simulink subsystem "PvtSubSys_HMI"  (R2020b)
settings: Solver=VariableStepAuto  StartTime=0.0  StopTime=10.0  RelTol=1e-3
undefined symbols (not defined in the file): P_HMI_LDW_LKAWarnTime, P_HMI_ObjectTypeFilter, P_HMI_WarnFormLDWReq
libraries: simulink x212, TrueDurationTime x6
(part 5 of 8)

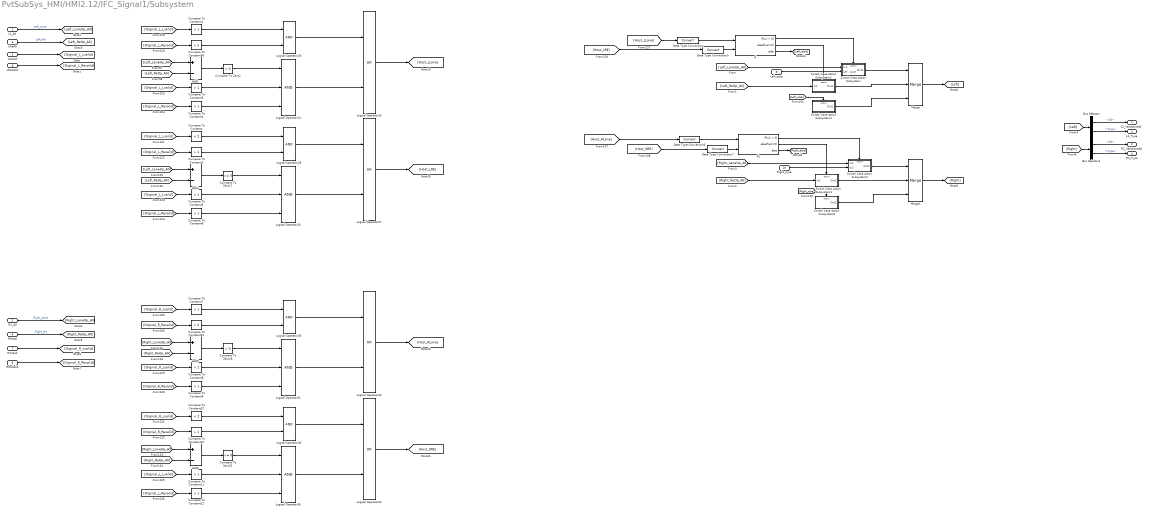
== system PvtSubSys_HMI/HMI2.12/IFC_Signal1/Subsystem ==
  L2_A0 : Inport
  R2_A0 : Inport  Port=2
  LReA0 : Inport  Port=3
  RReA0 : Inport  Port=4
  L2Valid : Inport  Port=5
  LReValid : Inport  Port=6
  R2Valid : Inport  Port=7
  RReValid : Inport  Port=8
  Left_type : Inport  Port=9
  Right_type : Inport  Port=10
  Add{1,4..6} (4 alike) : Sum  Inputs=+-
  Bus Selector : BusSelector  OutputSignals=A0,Type
  Bus Selector1 : BusSelector  OutputSignals=A0,Type
  Compare To Constant{,23,37..38} (4 alike) : simulink/Logic and Bit Operations/Compare To Constant  relop=<  const=2  OutDataTypeStr=boolean
  Compare To Constant{1..12} (12 alike) : simulink/Logic and Bit Operations/Compare To Constant  relop=>  const=1  OutDataTypeStr=boolean
  Compare To Zero17 : simulink/Logic and Bit Operations/Compare To Zero  relop=>=  OutDataTypeStr=boolean
  Compare To Zero2 : simulink/Logic and Bit Operations/Compare To Zero  relop=<  OutDataTypeStr=boolean
  Compare To Zero23 : simulink/Logic and Bit Operations/Compare To Zero  relop=<=  OutDataTypeStr=boolean
  Compare To Zero26 : simulink/Logic and Bit Operations/Compare To Zero  relop=>  OutDataTypeStr=boolean
  Data Type Conversion{,5..7} (4 alike) : DataTypeConversion
  If : If  NumInputs=2  ElseIfExpressions=u2>0
  If1 : If  NumInputs=2  ElseIfExpressions=u2>0
  Logical Operator{24,30..31,36} (4 alike) : Logic  Inputs=3  AllPortsSameDT=off  OutDataTypeStr=boolean
  Logical Operator{25,27,32..33} (4 alike) : Logic  Operator=OR  AllPortsSameDT=off  OutDataTypeStr=boolean
  Logical Operator{28..29,34..35} (4 alike) : Logic  AllPortsSameDT=off  OutDataTypeStr=boolean
  Merge : Merge  Inputs=3
  Merge1 : Merge  Inputs=3
  Switch Case Action Subsystem : Subsystem  TreatAsAtomicUnit=on
  Switch Case Action Subsystem1 : Subsystem  TreatAsAtomicUnit=on
  Switch Case Action Subsystem2 : Subsystem  TreatAsAtomicUnit=on
  Switch Case Action Subsystem3 : Subsystem  TreatAsAtomicUnit=on
  Switch Case Action Subsystem4 : Subsystem  TreatAsAtomicUnit=on
  Switch Case Action Subsystem5 : Subsystem  TreatAsAtomicUnit=on
  L2_ValidLaneA0 : Outport
  R2_ValidLaneA0 : Outport  Port=2
  L2_Type : Outport  Port=3
  R2_Type : Outport  Port=4
  wires:
  Bus Selector1/1 -> R2_ValidLaneA0/1  "<A0>"
  Bus Selector1/2 -> R2_Type/1  "<Type>"
  [Right] -> Bus Selector1/1
  Bus Selector/2 -> L2_Type/1  "<Type>"
  Bus Selector/1 -> L2_ValidLaneA0/1  "<A0>"
  [Left] -> Bus Selector/1
  Logical Operator33/1 -> [Host_RRE]
  Compare To Constant7/1 -> Logical Operator35/1
  Add5/1 -> Compare To Zero26/1
  Compare To Constant37/1 -> Logical Operator34/1
  [Orginal_L_Lvalid] -> Compare To Constant/1
  [Orginal_R_Lvalid] -> Compare To Constant7/1
  Compare To Constant3/1 -> Logical Operator24/2
  [Orginal_L_Revalid] -> Compare To Constant12/1
  Compare To Constant9/1 -> Logical Operator31/3
  Add6/1 -> Compare To Zero23/1
  Compare To Constant6/1 -> Logical Operator30/3
  Compare To Constant38/1 -> Logical Operator29/2
  Logical Operator32/1 -> [Host_RLane]
  Compare To Constant23/1 -> Logical Operator35/2
  Compare To Constant/1 -> Logical Operator28/1
  [Orginal_R_Lvalid] -> Compare To Constant8/1
  Logical Operator31/1 -> Logical Operator32/2
  [Right_LaneOp_A0] -> Add5/1
  Logical Operator34/1 -> Logical Operator33/1
  [Orginal_R_Revalid] -> Compare To Constant23/1
  [Right_ReOp_A0] -> Add6/2
  Logical Operator36/1 -> Logical Operator33/2
  [Right_LaneOp_A0] -> Add6/1
  [Orginal_R_Lvalid] -> Compare To Constant37/1
  [Orginal_L_Lvalid] -> Compare To Constant11/1
  [Orginal_R_Revalid] -> Compare To Constant9/1
  Compare To Constant11/1 -> Logical Operator36/2
  Compare To Constant12/1 -> Logical Operator36/3
  Compare To Constant10/1 -> Logical Operator34/2
  [Orginal_R_Revalid] -> Compare To Constant10/1
  Compare To Constant1/1 -> Logical Operator29/1
  [Left_LaneOp_A0] -> Add1/1
  Compare To Constant5/1 -> Logical Operator30/2
  Logical Operator27/1 -> [Host_LRE]
  Compare To Zero23/1 -> Logical Operator36/1
  Compare To Zero17/1 -> Logical Operator30/1
  Compare To Constant8/1 -> Logical Operator31/2
  [Orginal_L_Revalid] -> Compare To Constant2/1
  [Right_ReOp_A0] -> Add5/2
  Logical Operator25/1 -> [Host_LLane]
  Compare To Constant2/1 -> Logical Operator28/2
  Logical Operator30/1 -> Logical Operator27/2
  Logical Operator35/1 -> Logical Operator32/1
  [Orginal_L_Lvalid] -> Compare To Constant1/1
  [Orginal_L_Revalid] -> Compare To Constant6/1
  Logical Operator28/1 -> Logical Operator27/1
  Compare To Zero26/1 -> Logical Operator31/1
  [Orginal_L_Revalid] -> Compare To Constant38/1
  Add4/1 -> Compare To Zero17/1
  [Left_ReOp_A0] -> Add4/2
  [Left_LaneOp_A0] -> Add4/1
  Logical Operator24/1 -> Logical Operator25/2
  Logical Operator29/1 -> Logical Operator25/1
  [Orginal_L_Revalid] -> Compare To Constant4/1
  Add1/1 -> Compare To Zero2/1
  [Left_ReOp_A0] -> Add1/2
  [Orginal_L_Lvalid] -> Compare To Constant5/1
  Compare To Zero2/1 -> Logical Operator24/1
  [Orginal_L_Lvalid] -> Compare To Constant3/1
  Compare To Constant4/1 -> Logical Operator24/3
  Switch Case Action Subsystem5/1(Out1) -> Merge1/3
  If1/1 -> Switch Case Action Subsystem2/Action
  [Host_RLane] -> Data Type Conversion6/1
  Switch Case Action Subsystem4/1(Out1) -> Merge/3
  Data Type Conversion7/1 -> If1/2
  [Host_LLane] -> Data Type Conversion/1
  Switch Case Action Subsystem3/1(Out1) -> Merge1/2
  Switch Case Action Subsystem1/1(Out1) -> Merge/2
  If1/2 -> Switch Case Action Subsystem3/Action
  Switch Case Action Subsystem2/1(Out1) -> Merge1/1
  Data Type Conversion/1 -> If/1
  [Host_LRE] -> Data Type Conversion5/1
  If/3 -> [Left_else]
  [Host_RRE] -> Data Type Conversion7/1
  [Right_else] -> Switch Case Action Subsystem5/Action
  Switch Case Action Subsystem/1(Out1) -> Merge/1
  Data Type Conversion6/1 -> If1/1
  If/2 -> Switch Case Action Subsystem1/Action
  If/1 -> Switch Case Action Subsystem/Action
  Data Type Conversion5/1 -> If/2
  If1/3 -> [Right_else]
  [Left_else] -> Switch Case Action Subsystem4/Action
  L2Valid/1 -> [Orginal_L_Lvalid]
  LReValid/1 -> [Orginal_L_Revalid]
  L2_A0/1 -> [Left_LaneOp_A0]  "Left_Lane"
  LReA0/1 -> [Left_ReOp_A0]  "Left_Re"
  R2_A0/1 -> [Right_LaneOp_A0]  "Right_Lane"
  RReA0/1 -> [Right_ReOp_A0]  "Right_Re"
  R2Valid/1 -> [Orginal_R_Lvalid]
  RReValid/1 -> [Orginal_R_Revalid]
  [Left_LaneOp_A0] -> Switch Case Action Subsystem/1(In1)
  [Left_ReOp_A0] -> Switch Case Action Subsystem1/1(In1)
  [Right_LaneOp_A0] -> Switch Case Action Subsystem2/1(In1)
  [Right_ReOp_A0] -> Switch Case Action Subsystem3/1(In1)
  Merge/1 -> [Left]
  Merge1/1 -> [Right]
  Left_type/1 -> Switch Case Action Subsystem/2(Left_type)
  Right_type/1 -> Switch Case Action Subsystem2/2(In2)

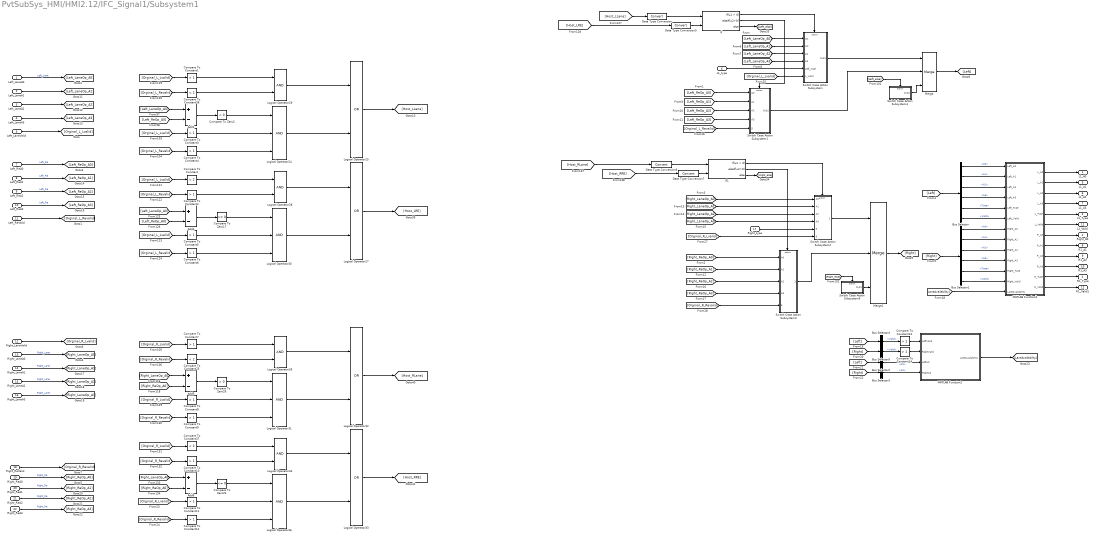
== system PvtSubSys_HMI/HMI2.12/IFC_Signal1/Subsystem1 ==
  Left_LaneA0 : Inport
  Left_LaneA1 : Inport  Port=2
  Left_LaneA2 : Inport  Port=3
  Left_LaneA3 : Inport  Port=4
  Left_LaneValid : Inport  Port=5
  L1_type : Inport  Port=6
  Left_ReA0 : Inport  Port=7
  Left_ReA1 : Inport  Port=8
  Left_ReA2 : Inport  Port=9
  Left_ReA3 : Inport  Port=10
  Left_ReValid : Inport  Port=11
  Right_LaneValid : Inport  Port=12
  Right_LaneA0 : Inport  Port=13
  Right_LaneA1 : Inport  Port=14
  Right_LaneA2 : Inport  Port=15
  Right_LaneA3 : Inport  Port=16
  Right_type : Inport  Port=17
  Right_ReValid : Inport  Port=18
  Right_ReA0 : Inport  Port=19
  Right_ReA1 : Inport  Port=20
  Right_ReA2 : Inport  Port=21
  Right_ReA3 : Inport  Port=22
  Add{1,4..6} (4 alike) : Sum  Inputs=+-
  Bus Selector : BusSelector  OutputSignals=A0,A1,A2,A3,Type,Valid
  Bus Selector1 : BusSelector  OutputSignals=A0,A1,A2,A3,Type,Valid
  Bus Selector2 : BusSelector  OutputSignals=A0
  Bus Selector3 : BusSelector  OutputSignals=A0
  Bus Selector4 : BusSelector  OutputSignals=Valid
  Bus Selector5 : BusSelector  OutputSignals=Valid
  Compare To Constant{,23,37..38} (4 alike) : simulink/Logic and Bit Operations/Compare To Constant  relop=<  const=2  OutDataTypeStr=boolean
  Compare To Constant{1..14} (14 alike) : simulink/Logic and Bit Operations/Compare To Constant  relop=>  const=1  OutDataTypeStr=boolean
  Compare To Zero17 : simulink/Logic and Bit Operations/Compare To Zero  relop=>=  OutDataTypeStr=boolean
  Compare To Zero2 : simulink/Logic and Bit Operations/Compare To Zero  relop=<  OutDataTypeStr=boolean
  Compare To Zero23 : simulink/Logic and Bit Operations/Compare To Zero  relop=<=  OutDataTypeStr=boolean
  Compare To Zero26 : simulink/Logic and Bit Operations/Compare To Zero  relop=>  OutDataTypeStr=boolean
  Data Type Conversion{,5..7} (4 alike) : DataTypeConversion
  If : If  NumInputs=2  ElseIfExpressions=u2>0
  If1 : If  NumInputs=2  ElseIfExpressions=u2>0
  Logical Operator{24,30..31,36} (4 alike) : Logic  Inputs=3  AllPortsSameDT=off  OutDataTypeStr=boolean
  Logical Operator{25,27,32..33} (4 alike) : Logic  Operator=OR  AllPortsSameDT=off  OutDataTypeStr=boolean
  Logical Operator{28..29,34..35} (4 alike) : Logic  AllPortsSameDT=off  OutDataTypeStr=boolean
  MATLAB Function2 : MATLAB Function  TreatAsAtomicUnit=on
  MATLAB Function3 : MATLAB Function  TreatAsAtomicUnit=on
  Merge : Merge  Inputs=3
  Merge1 : Merge  Inputs=3
  Switch Case Action Subsystem : Subsystem  TreatAsAtomicUnit=on
  Switch Case Action Subsystem1 : Subsystem  TreatAsAtomicUnit=on
  Switch Case Action Subsystem2 : Subsystem  TreatAsAtomicUnit=on
  Switch Case Action Subsystem3 : Subsystem  TreatAsAtomicUnit=on
  Switch Case Action Subsystem4 : Subsystem  TreatAsAtomicUnit=on
  Switch Case Action Subsystem5 : Subsystem  TreatAsAtomicUnit=on
  L1_A0 : Outport
  Right_A0 : Outport  Port=2
  L1_Type : Outport  Port=3
  R1_Type : Outport  Port=4
  L1_A1 : Outport  Port=5
  L1_A2 : Outport  Port=6
  L1_A3 : Outport  Port=7
  R1_A1 : Outport  Port=8
  R1_A2 : Outport  Port=9
  R1_A3 : Outport  Port=10
  L1_Valid : Outport  Port=11
  R1_Valid1 : Outport  Port=12
  wires:
  Bus Selector1/6 -> MATLAB Function3/12(Right_Valid)  "<Valid>"
  [Orginal_R_Revalid] -> Switch Case Action Subsystem3/5(Valid)
  [Orginal_R_Lvalid] -> Switch Case Action Subsystem2/6(Valid)
  [Orginal_L_Revalid] -> Switch Case Action Subsystem1/5(LRE_Valid)
  [Orginal_L_Lvalid] -> Switch Case Action Subsystem/6(L_Valid)
  Bus Selector/6 -> MATLAB Function3/6(Left_Valid)  "<Valid>"
  Compare To Constant14/1 -> MATLAB Function2/2(RightValid)
  Bus Selector5/1 -> Compare To Constant14/1  "<Valid>"
  [Right] -> Bus Selector5/1
  Compare To Constant13/1 -> MATLAB Function2/1(LeftValid)
  Bus Selector4/1 -> Compare To Constant13/1  "<Valid>"
  [Left] -> Bus Selector4/1
  Bus Selector3/1 -> MATLAB Function2/4(RightA0)  "<A0>"
  [Right] -> Bus Selector3/1
  Bus Selector2/1 -> MATLAB Function2/3(LeftA0)  "<A0>"
  [Left] -> Bus Selector2/1
  MATLAB Function3/12(R_Valid) -> R1_Valid1/1
  MATLAB Function3/6(L_Valid) -> L1_Valid/1
  MATLAB Function2/1(LaneAvailability) -> [LaneAvailability]
  MATLAB Function3/10(R_A3) -> R1_A3/1
  MATLAB Function3/9(R_A2) -> R1_A2/1
  MATLAB Function3/8(R_A1) -> R1_A1/1
  MATLAB Function3/4(L_A3) -> L1_A3/1
  MATLAB Function3/3(L_A2) -> L1_A2/1
  MATLAB Function3/2(L_A1) -> L1_A1/1
  Bus Selector1/4 -> MATLAB Function3/10(Right_A3)  "<A3>"
  Bus Selector1/3 -> MATLAB Function3/9(Right_A2)  "<A2>"
  Bus Selector1/2 -> MATLAB Function3/8(Right_A1)  "<A1>"
  Bus Selector/4 -> MATLAB Function3/4(Left_A3)  "<A3>"
  Bus Selector/3 -> MATLAB Function3/3(Left_A2)  "<A2>"
  Bus Selector/2 -> MATLAB Function3/2(Left_A1)  "<A1>"
  [Right_ReOp_A3] -> Switch Case Action Subsystem3/4(A3)
  [Right_ReOp_A2] -> Switch Case Action Subsystem3/3(A2)
  [Right_ReOp_A1] -> Switch Case Action Subsystem3/2(A1)
  [Right_LaneOp_A3] -> Switch Case Action Subsystem2/4(A3)
  [Right_LaneOp_A2] -> Switch Case Action Subsystem2/3(A2)
  [Right_LaneOp_A1] -> Switch Case Action Subsystem2/2(A1)
  Right_type/1 -> Switch Case Action Subsystem2/5(Right_type)
  [Left_ReOp_A3] -> Switch Case Action Subsystem1/4(A3)
  [Left_ReOp_A2] -> Switch Case Action Subsystem1/3(A2)
  [Left_ReOp_A1] -> Switch Case Action Subsystem1/2(A1)
  [Left_LaneOp_A3] -> Switch Case Action Subsystem/4(A3)
  [Left_LaneOp_A2] -> Switch Case Action Subsystem/3(A2)
  [Left_LaneOp_A1] -> Switch Case Action Subsystem/2(In2)
  L1_type/1 -> Switch Case Action Subsystem/5(Left_type)
  Right_ReA1/1 -> [Right_ReOp_A1]  "Right_Re"
  Right_ReA2/1 -> [Right_ReOp_A2]  "Right_Re"
  Right_ReA3/1 -> [Right_ReOp_A3]  "Right_Re"
  Right_LaneA3/1 -> [Right_LaneOp_A3]  "Right_Lane"
  Right_LaneA2/1 -> [Right_LaneOp_A2]  "Right_Lane"
  Right_LaneA1/1 -> [Right_LaneOp_A1]  "Right_Lane"
  Left_ReA1/1 -> [Left_ReOp_A1]  "Left_Re"
  Left_ReA2/1 -> [Left_ReOp_A2]  "Left_Re"
  Left_ReA3/1 -> [Left_ReOp_A3]  "Left_Re"
  Left_LaneA3/1 -> [Left_LaneOp_A3]
  Left_LaneA2/1 -> [Left_LaneOp_A2]
  Left_LaneA1/1 -> [Left_LaneOp_A1]
  Logical Operator33/1 -> [Host_RRE]
  Compare To Constant7/1 -> Logical Operator35/1
  Add5/1 -> Compare To Zero26/1
  Compare To Constant37/1 -> Logical Operator34/1
  [Orginal_L_Lvalid] -> Compare To Constant/1
  [Orginal_R_Lvalid] -> Compare To Constant7/1
  Compare To Constant3/1 -> Logical Operator24/2
  [Orginal_R_Revalid] -> Compare To Constant12/1
  Compare To Constant9/1 -> Logical Operator31/3
  Add6/1 -> Compare To Zero23/1
  Compare To Constant6/1 -> Logical Operator30/3
  Compare To Constant38/1 -> Logical Operator29/2
  Logical Operator32/1 -> [Host_RLane]
  Compare To Constant23/1 -> Logical Operator35/2
  Compare To Constant/1 -> Logical Operator28/1
  [Orginal_R_Lvalid] -> Compare To Constant8/1
  Logical Operator31/1 -> Logical Operator32/2
  [Right_LaneOp_A0] -> Add5/1
  Logical Operator34/1 -> Logical Operator33/1
  [Orginal_R_Revalid] -> Compare To Constant23/1
  [Right_ReOp_A0] -> Add6/2
  Logical Operator36/1 -> Logical Operator33/2
  [Right_LaneOp_A0] -> Add6/1
  [Orginal_R_Lvalid] -> Compare To Constant37/1
  [Orginal_R_Lvalid] -> Compare To Constant11/1
  [Orginal_R_Revalid] -> Compare To Constant9/1
  Compare To Constant11/1 -> Logical Operator36/2
  Compare To Constant12/1 -> Logical Operator36/3
  Compare To Constant10/1 -> Logical Operator34/2
  [Orginal_R_Revalid] -> Compare To Constant10/1
  Compare To Constant1/1 -> Logical Operator29/1
  [Left_LaneOp_A0] -> Add1/1
  Compare To Constant5/1 -> Logical Operator30/2
  Logical Operator27/1 -> [Host_LRE]
  Compare To Zero23/1 -> Logical Operator36/1
  Compare To Zero17/1 -> Logical Operator30/1
  Compare To Constant8/1 -> Logical Operator31/2
  [Orginal_L_Revalid] -> Compare To Constant2/1
  [Right_ReOp_A0] -> Add5/2
  Logical Operator25/1 -> [Host_LLane]
  Compare To Constant2/1 -> Logical Operator28/2
  Logical Operator30/1 -> Logical Operator27/2
  Logical Operator35/1 -> Logical Operator32/1
  [Orginal_L_Lvalid] -> Compare To Constant1/1
  [Orginal_L_Revalid] -> Compare To Constant6/1
  Logical Operator28/1 -> Logical Operator27/1
  Compare To Zero26/1 -> Logical Operator31/1
  [Orginal_L_Revalid] -> Compare To Constant38/1
  Add4/1 -> Compare To Zero17/1
  [Left_ReOp_A0] -> Add4/2
  [Left_LaneOp_A0] -> Add4/1
  Logical Operator24/1 -> Logical Operator25/2
  Logical Operator29/1 -> Logical Operator25/1
  [Orginal_L_Revalid] -> Compare To Constant4/1
  Add1/1 -> Compare To Zero2/1
  [Left_ReOp_A0] -> Add1/2
  [Orginal_L_Lvalid] -> Compare To Constant5/1
  Compare To Zero2/1 -> Logical Operator24/1
  [Orginal_L_Lvalid] -> Compare To Constant3/1
  Compare To Constant4/1 -> Logical Operator24/3
  Switch Case Action Subsystem5/1(Out1) -> Merge1/3
  If1/1 -> Switch Case Action Subsystem2/Action
  [Host_RLane] -> Data Type Conversion6/1
  Switch Case Action Subsystem4/1(Out2) -> Merge/3
  Data Type Conversion7/1 -> If1/2
  [Host_LLane] -> Data Type Conversion/1
  Switch Case Action Subsystem3/1(Out1) -> Merge1/2
  Switch Case Action Subsystem1/1(Out2) -> Merge/2
  If1/2 -> Switch Case Action Subsystem3/Action
  Switch Case Action Subsystem2/1(Out1) -> Merge1/1
  Data Type Conversion/1 -> If/1
  [Host_LRE] -> Data Type Conversion5/1
  If/3 -> [Left_else]
  [Host_RRE] -> Data Type Conversion7/1
  [Right_else] -> Switch Case Action Subsystem5/Action
  Switch Case Action Subsystem/1(Out1) -> Merge/1
  Data Type Conversion6/1 -> If1/1
  If/2 -> Switch Case Action Subsystem1/Action
  If/1 -> Switch Case Action Subsystem/Action
  Data Type Conversion5/1 -> If/2
  If1/3 -> [Right_else]
  [Left_else] -> Switch Case Action Subsystem4/Action
  Left_LaneValid/1 -> [Orginal_L_Lvalid]
  Left_ReValid/1 -> [Orginal_L_Revalid]
  Left_LaneA0/1 -> [Left_LaneOp_A0]  "Left_Lane"
  Left_ReA0/1 -> [Left_ReOp_A0]  "Left_Re"
  Right_LaneA0/1 -> [Right_LaneOp_A0]  "Right_Lane"
  Right_ReA0/1 -> [Right_ReOp_A0]  "Right_Re"
  Right_LaneValid/1 -> [Orginal_R_Lvalid]
  Right_ReValid/1 -> [Orginal_R_Revalid]
  [Left_LaneOp_A0] -> Switch Case Action Subsystem/1(In1)
  [Left_ReOp_A0] -> Switch Case Action Subsystem1/1(A0)
  [Right_LaneOp_A0] -> Switch Case Action Subsystem2/1(A0)
  [Right_ReOp_A0] -> Switch Case Action Subsystem3/1(A0)
  MATLAB Function3/1(L_A0) -> L1_A0/1
  Merge/1 -> [Left]
  [Left] -> Bus Selector/1
  Merge1/1 -> [Right]
  [Right] -> Bus Selector1/1
  [LaneAvailability] -> MATLAB Function3/13(LaneAvailability)
  Bus Selector/1 -> MATLAB Function3/1(Left_A0)  "<A0>"
  Bus Selector/5 -> MATLAB Function3/5(Left_Type)  "<Type>"
  Bus Selector1/1 -> MATLAB Function3/7(Right_A0)  "<A0>"
  Bus Selector1/5 -> MATLAB Function3/11(Right_Type)  "<Type>"
  MATLAB Function3/7(R_A0) -> Right_A0/1
  MATLAB Function3/11(R_Type) -> R1_Type/1
  MATLAB Function3/5(L_Type) -> L1_Type/1

== system PvtSubSys_HMI/HMI2.12/IFC_Signal1/Subsystem10 ==
  note: When the vehicle stops, stop updating
  note: 存在一帧丢失状况
  standstill : Inport
  in : Inport  Port=2
  Compare To Constant10 : simulink/Logic and Bit Operations/Compare To Constant  relop===  const=1  OutDataTypeStr=boolean
  Compare To Constant9 : simulink/Logic and Bit Operations/Compare To Constant  relop===  const=0  OutDataTypeStr=boolean
  Logical Operator8 : Logic  AllPortsSameDT=off  OutDataTypeStr=boolean
  MATLAB Function1 : MATLAB Function  TreatAsAtomicUnit=on
  Unit Delay : UnitDelay  SampleTime=-1  HasFrameUpgradeWarning=on
  Unit Delay3 : UnitDelay  SampleTime=-1  HasFrameUpgradeWarning=on
  out : Outport
  wires:
  Logical Operator8/1 -> MATLAB Function1/3(update)
  standstill/1 -> MATLAB Function1/1(standstill), Compare To Constant10/1, Unit Delay3/1
  Compare To Constant9/1 -> Logical Operator8/1
  in/1 -> MATLAB Function1/2(in)
  MATLAB Function1/2(recorder) -> Unit Delay/1
  Unit Delay3/1 -> Compare To Constant9/1
  Compare To Constant10/1 -> Logical Operator8/2
  Unit Delay/1 -> MATLAB Function1/4(inrecorder)
  MATLAB Function1/1(out) -> out/1

== system PvtSubSys_HMI/HMI2.12/IFC_Signal1/Subsystem11 ==
  note: When the vehicle stops, stop updating
  note: 存在一帧丢失状况
  standstill : Inport
  in : Inport  Port=2
  Compare To Constant10 : simulink/Logic and Bit Operations/Compare To Constant  relop===  const=1  OutDataTypeStr=boolean
  Compare To Constant9 : simulink/Logic and Bit Operations/Compare To Constant  relop===  const=0  OutDataTypeStr=boolean
  Logical Operator8 : Logic  AllPortsSameDT=off  OutDataTypeStr=boolean
  MATLAB Function1 : MATLAB Function  TreatAsAtomicUnit=on
  Unit Delay : UnitDelay  SampleTime=-1  HasFrameUpgradeWarning=on
  Unit Delay3 : UnitDelay  SampleTime=-1  HasFrameUpgradeWarning=on
  out : Outport
  wires:
  Logical Operator8/1 -> MATLAB Function1/3(update)
  standstill/1 -> MATLAB Function1/1(standstill), Compare To Constant10/1, Unit Delay3/1
  Compare To Constant9/1 -> Logical Operator8/1
  in/1 -> MATLAB Function1/2(in)
  MATLAB Function1/2(recorder) -> Unit Delay/1
  Unit Delay3/1 -> Compare To Constant9/1
  Compare To Constant10/1 -> Logical Operator8/2
  Unit Delay/1 -> MATLAB Function1/4(inrecorder)
  MATLAB Function1/1(out) -> out/1

== system PvtSubSys_HMI/HMI2.12/IFC_Signal1/Subsystem12 ==
  note: 存在一帧丢失状况
  note: When the vehicle stops, stop updating
  standstill : Inport
  in : Inport  Port=2
  Compare To Constant10 : simulink/Logic and Bit Operations/Compare To Constant  relop===  const=1  OutDataTypeStr=boolean
  Compare To Constant9 : simulink/Logic and Bit Operations/Compare To Constant  relop===  const=0  OutDataTypeStr=boolean
  Logical Operator8 : Logic  AllPortsSameDT=off  OutDataTypeStr=boolean
  MATLAB Function1 : MATLAB Function  TreatAsAtomicUnit=on
  Unit Delay : UnitDelay  SampleTime=-1  HasFrameUpgradeWarning=on
  Unit Delay3 : UnitDelay  SampleTime=-1  HasFrameUpgradeWarning=on
  out : Outport
  wires:
  MATLAB Function1/1(out) -> out/1
  Unit Delay/1 -> MATLAB Function1/4(inrecorder)
  Compare To Constant10/1 -> Logical Operator8/2
  Unit Delay3/1 -> Compare To Constant9/1
  MATLAB Function1/2(recorder) -> Unit Delay/1
  in/1 -> MATLAB Function1/2(in)
  Compare To Constant9/1 -> Logical Operator8/1
  standstill/1 -> Unit Delay3/1, Compare To Constant10/1, MATLAB Function1/1(standstill)
  Logical Operator8/1 -> MATLAB Function1/3(update)

== system PvtSubSys_HMI/HMI2.12/IFC_Signal1/Subsystem13 ==
  note: When the vehicle stops, stop updating
  note: 存在一帧丢失状况
  standstill : Inport
  in : Inport  Port=2
  Compare To Constant10 : simulink/Logic and Bit Operations/Compare To Constant  relop===  const=1  OutDataTypeStr=boolean
  Compare To Constant9 : simulink/Logic and Bit Operations/Compare To Constant  relop===  const=0  OutDataTypeStr=boolean
  Logical Operator8 : Logic  AllPortsSameDT=off  OutDataTypeStr=boolean
  MATLAB Function1 : MATLAB Function  TreatAsAtomicUnit=on
  Unit Delay : UnitDelay  SampleTime=-1  HasFrameUpgradeWarning=on
  Unit Delay3 : UnitDelay  SampleTime=-1  HasFrameUpgradeWarning=on
  out : Outport
  wires:
  Logical Operator8/1 -> MATLAB Function1/3(update)
  standstill/1 -> MATLAB Function1/1(standstill), Compare To Constant10/1, Unit Delay3/1
  Compare To Constant9/1 -> Logical Operator8/1
  in/1 -> MATLAB Function1/2(in)
  MATLAB Function1/2(recorder) -> Unit Delay/1
  Unit Delay3/1 -> Compare To Constant9/1
  Compare To Constant10/1 -> Logical Operator8/2
  Unit Delay/1 -> MATLAB Function1/4(inrecorder)
  MATLAB Function1/1(out) -> out/1

== system PvtSubSys_HMI/HMI2.12/IFC_Signal1/Subsystem14 ==
  note: 存在一帧丢失状况
  note: When the vehicle stops, stop updating
  standstill : Inport
  in : Inport  Port=2
  Compare To Constant10 : simulink/Logic and Bit Operations/Compare To Constant  relop===  const=1  OutDataTypeStr=boolean
  Compare To Constant9 : simulink/Logic and Bit Operations/Compare To Constant  relop===  const=0  OutDataTypeStr=boolean
  Logical Operator8 : Logic  AllPortsSameDT=off  OutDataTypeStr=boolean
  MATLAB Function1 : MATLAB Function  TreatAsAtomicUnit=on
  Unit Delay : UnitDelay  SampleTime=-1  HasFrameUpgradeWarning=on
  Unit Delay3 : UnitDelay  SampleTime=-1  HasFrameUpgradeWarning=on
  out : Outport
  wires:
  MATLAB Function1/1(out) -> out/1
  Unit Delay/1 -> MATLAB Function1/4(inrecorder)
  Compare To Constant10/1 -> Logical Operator8/2
  Unit Delay3/1 -> Compare To Constant9/1
  MATLAB Function1/2(recorder) -> Unit Delay/1
  in/1 -> MATLAB Function1/2(in)
  Compare To Constant9/1 -> Logical Operator8/1
  standstill/1 -> Unit Delay3/1, Compare To Constant10/1, MATLAB Function1/1(standstill)
  Logical Operator8/1 -> MATLAB Function1/3(update)

== system PvtSubSys_HMI/HMI2.12/IFC_Signal1/Subsystem15 ==
  note: When the vehicle stops, stop updating
  note: 存在一帧丢失状况
  standstill : Inport
  in : Inport  Port=2
  Compare To Constant10 : simulink/Logic and Bit Operations/Compare To Constant  relop===  const=1  OutDataTypeStr=boolean
  Compare To Constant9 : simulink/Logic and Bit Operations/Compare To Constant  relop===  const=0  OutDataTypeStr=boolean
  Logical Operator8 : Logic  AllPortsSameDT=off  OutDataTypeStr=boolean
  MATLAB Function1 : MATLAB Function  TreatAsAtomicUnit=on
  Unit Delay : UnitDelay  SampleTime=-1  HasFrameUpgradeWarning=on
  Unit Delay3 : UnitDelay  SampleTime=-1  HasFrameUpgradeWarning=on
  out : Outport
  wires:
  Logical Operator8/1 -> MATLAB Function1/3(update)
  standstill/1 -> MATLAB Function1/1(standstill), Compare To Constant10/1, Unit Delay3/1
  Compare To Constant9/1 -> Logical Operator8/1
  in/1 -> MATLAB Function1/2(in)
  MATLAB Function1/2(recorder) -> Unit Delay/1
  Unit Delay3/1 -> Compare To Constant9/1
  Compare To Constant10/1 -> Logical Operator8/2
  Unit Delay/1 -> MATLAB Function1/4(inrecorder)
  MATLAB Function1/1(out) -> out/1

== system PvtSubSys_HMI/HMI2.12/IFC_Signal1/Subsystem16 ==
  note: 存在一帧丢失状况
  note: When the vehicle stops, stop updating
  standstill : Inport
  in : Inport  Port=2
  Compare To Constant10 : simulink/Logic and Bit Operations/Compare To Constant  relop===  const=1  OutDataTypeStr=boolean
  Compare To Constant9 : simulink/Logic and Bit Operations/Compare To Constant  relop===  const=0  OutDataTypeStr=boolean
  Logical Operator8 : Logic  AllPortsSameDT=off  OutDataTypeStr=boolean
  MATLAB Function1 : MATLAB Function  TreatAsAtomicUnit=on
  Unit Delay : UnitDelay  SampleTime=-1  HasFrameUpgradeWarning=on
  Unit Delay3 : UnitDelay  SampleTime=-1  HasFrameUpgradeWarning=on
  out : Outport
  wires:
  MATLAB Function1/1(out) -> out/1
  Unit Delay/1 -> MATLAB Function1/4(inrecorder)
  Compare To Constant10/1 -> Logical Operator8/2
  Unit Delay3/1 -> Compare To Constant9/1
  MATLAB Function1/2(recorder) -> Unit Delay/1
  in/1 -> MATLAB Function1/2(in)
  Compare To Constant9/1 -> Logical Operator8/1
  standstill/1 -> Unit Delay3/1, Compare To Constant10/1, MATLAB Function1/1(standstill)
  Logical Operator8/1 -> MATLAB Function1/3(update)

== system PvtSubSys_HMI/HMI2.12/IFC_Signal1/Subsystem17 ==
  note: 存在一帧丢失状况
  note: When the vehicle stops, stop updating
  standstill : Inport
  in : Inport  Port=2
  Compare To Constant10 : simulink/Logic and Bit Operations/Compare To Constant  relop===  const=1  OutDataTypeStr=boolean
  Compare To Constant9 : simulink/Logic and Bit Operations/Compare To Constant  relop===  const=0  OutDataTypeStr=boolean
  Logical Operator8 : Logic  AllPortsSameDT=off  OutDataTypeStr=boolean
  MATLAB Function1 : MATLAB Function  TreatAsAtomicUnit=on
  Unit Delay : UnitDelay  SampleTime=-1  HasFrameUpgradeWarning=on
  Unit Delay3 : UnitDelay  SampleTime=-1  HasFrameUpgradeWarning=on
  out : Outport
  wires:
  MATLAB Function1/1(out) -> out/1
  Unit Delay/1 -> MATLAB Function1/4(inrecorder)
  Compare To Constant10/1 -> Logical Operator8/2
  Unit Delay3/1 -> Compare To Constant9/1
  MATLAB Function1/2(recorder) -> Unit Delay/1
  in/1 -> MATLAB Function1/2(in)
  Compare To Constant9/1 -> Logical Operator8/1
  standstill/1 -> Unit Delay3/1, Compare To Constant10/1, MATLAB Function1/1(standstill)
  Logical Operator8/1 -> MATLAB Function1/3(update)

== system PvtSubSys_HMI/HMI2.12/IFC_Signal1/Subsystem18 ==
  note: When the vehicle stops, stop updating
  note: 存在一帧丢失状况
  standstill : Inport
  in : Inport  Port=2
  Compare To Constant10 : simulink/Logic and Bit Operations/Compare To Constant  relop===  const=1  OutDataTypeStr=boolean
  Compare To Constant9 : simulink/Logic and Bit Operations/Compare To Constant  relop===  const=0  OutDataTypeStr=boolean
  Logical Operator8 : Logic  AllPortsSameDT=off  OutDataTypeStr=boolean
  MATLAB Function1 : MATLAB Function  TreatAsAtomicUnit=on
  Unit Delay : UnitDelay  SampleTime=-1  HasFrameUpgradeWarning=on
  Unit Delay3 : UnitDelay  SampleTime=-1  HasFrameUpgradeWarning=on
  out : Outport
  wires:
  Logical Operator8/1 -> MATLAB Function1/3(update)
  standstill/1 -> MATLAB Function1/1(standstill), Compare To Constant10/1, Unit Delay3/1
  Compare To Constant9/1 -> Logical Operator8/1
  in/1 -> MATLAB Function1/2(in)
  MATLAB Function1/2(recorder) -> Unit Delay/1
  Unit Delay3/1 -> Compare To Constant9/1
  Compare To Constant10/1 -> Logical Operator8/2
  Unit Delay/1 -> MATLAB Function1/4(inrecorder)
  MATLAB Function1/1(out) -> out/1

== system PvtSubSys_HMI/HMI2.12/IFC_Signal1/Subsystem19 ==
  note: 存在一帧丢失状况
  note: When the vehicle stops, stop updating
  standstill : Inport
  in : Inport  Port=2
  Compare To Constant10 : simulink/Logic and Bit Operations/Compare To Constant  relop===  const=1  OutDataTypeStr=boolean
  Compare To Constant9 : simulink/Logic and Bit Operations/Compare To Constant  relop===  const=0  OutDataTypeStr=boolean
  Logical Operator8 : Logic  AllPortsSameDT=off  OutDataTypeStr=boolean
  MATLAB Function1 : MATLAB Function  TreatAsAtomicUnit=on
  Unit Delay : UnitDelay  SampleTime=-1  HasFrameUpgradeWarning=on
  Unit Delay3 : UnitDelay  SampleTime=-1  HasFrameUpgradeWarning=on
  out : Outport
  wires:
  MATLAB Function1/1(out) -> out/1
  Unit Delay/1 -> MATLAB Function1/4(inrecorder)
  Compare To Constant10/1 -> Logical Operator8/2
  Unit Delay3/1 -> Compare To Constant9/1
  MATLAB Function1/2(recorder) -> Unit Delay/1
  in/1 -> MATLAB Function1/2(in)
  Compare To Constant9/1 -> Logical Operator8/1
  standstill/1 -> Unit Delay3/1, Compare To Constant10/1, MATLAB Function1/1(standstill)
  Logical Operator8/1 -> MATLAB Function1/3(update)

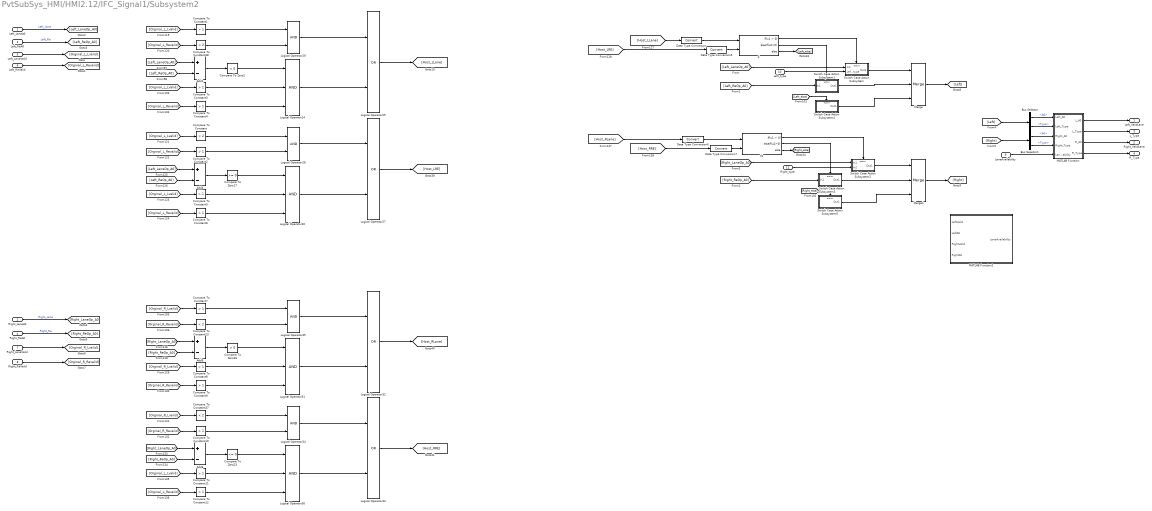
== system PvtSubSys_HMI/HMI2.12/IFC_Signal1/Subsystem2 ==
  Left_LaneA0 : Inport
  Right_LaneA0 : Inport  Port=2
  Left_ReA0 : Inport  Port=3
  Right_ReA0 : Inport  Port=4
  Left_LaneValid : Inport  Port=5
  Left_ReValid : Inport  Port=6
  Right_LaneValid : Inport  Port=7
  Right_ReValid : Inport  Port=8
  LaneAvailability : Inport  Port=9
  Left_type : Inport  Port=10
  Right_type : Inport  Port=11
  Add{1,4..6} (4 alike) : Sum  Inputs=+-
  Bus Selector : BusSelector  OutputSignals=A0,Type
  Bus Selector1 : BusSelector  OutputSignals=A0,Type
  Compare To Constant{,23,37..38} (4 alike) : simulink/Logic and Bit Operations/Compare To Constant  relop=<  const=2  OutDataTypeStr=boolean
  Compare To Constant{1..12} (12 alike) : simulink/Logic and Bit Operations/Compare To Constant  relop=>  const=1  OutDataTypeStr=boolean
  Compare To Zero17 : simulink/Logic and Bit Operations/Compare To Zero  relop=>=  OutDataTypeStr=boolean
  Compare To Zero2 : simulink/Logic and Bit Operations/Compare To Zero  relop=<  OutDataTypeStr=boolean
  Compare To Zero23 : simulink/Logic and Bit Operations/Compare To Zero  relop=<=  OutDataTypeStr=boolean
  Compare To Zero26 : simulink/Logic and Bit Operations/Compare To Zero  relop=>  OutDataTypeStr=boolean
  Data Type Conversion{,5..7} (4 alike) : DataTypeConversion
  If : If  NumInputs=2  ElseIfExpressions=u2>0
  If1 : If  NumInputs=2  ElseIfExpressions=u2>0
  Logical Operator{24,30..31,36} (4 alike) : Logic  Inputs=3  AllPortsSameDT=off  OutDataTypeStr=boolean
  Logical Operator{25,27,32..33} (4 alike) : Logic  Operator=OR  AllPortsSameDT=off  OutDataTypeStr=boolean
  Logical Operator{28..29,34..35} (4 alike) : Logic  AllPortsSameDT=off  OutDataTypeStr=boolean
  MATLAB Function : MATLAB Function  TreatAsAtomicUnit=on
  MATLAB Function2 : MATLAB Function  TreatAsAtomicUnit=on
  Merge : Merge  Inputs=3
  Merge1 : Merge  Inputs=3
  Switch Case Action Subsystem : Subsystem  TreatAsAtomicUnit=on
  Switch Case Action Subsystem1 : Subsystem  TreatAsAtomicUnit=on
  Switch Case Action Subsystem2 : Subsystem  TreatAsAtomicUnit=on
  Switch Case Action Subsystem3 : Subsystem  TreatAsAtomicUnit=on
  Switch Case Action Subsystem4 : Subsystem  TreatAsAtomicUnit=on
  Switch Case Action Subsystem5 : Subsystem  TreatAsAtomicUnit=on
  Left_ValidLane : Outport
  Right_ValidLane : Outport  Port=2
  L_Type : Outport  Port=3
  R_Type : Outport  Port=4
  wires:
  MATLAB Function/2(L_Type) -> L_Type/1
  MATLAB Function/4(R_Type) -> R_Type/1
  MATLAB Function/3(R_A0) -> Right_ValidLane/1
  Bus Selector1/2 -> MATLAB Function/4(Right_Type)  "<Type>"
  Bus Selector1/1 -> MATLAB Function/3(Right_A0)  "<A0>"
  Bus Selector/2 -> MATLAB Function/2(Left_Type)  "<Type>"
  Bus Selector/1 -> MATLAB Function/1(Left_A0)  "<A0>"
  Right_type/1 -> Switch Case Action Subsystem2/2(In2)
  Left_type/1 -> Switch Case Action Subsystem/2(Left_type)
  LaneAvailability/1 -> MATLAB Function/5(LaneAvailability)
  [Right] -> Bus Selector1/1
  Merge1/1 -> [Right]
  [Left] -> Bus Selector/1
  Merge/1 -> [Left]
  MATLAB Function/1(L_A0) -> Left_ValidLane/1
  [Right_ReOp_A0] -> Switch Case Action Subsystem3/1(In1)
  [Right_LaneOp_A0] -> Switch Case Action Subsystem2/1(In1)
  [Left_ReOp_A0] -> Switch Case Action Subsystem1/1(In1)
  [Left_LaneOp_A0] -> Switch Case Action Subsystem/1(In1)
  Right_ReValid/1 -> [Orginal_R_Revalid]
  Right_LaneValid/1 -> [Orginal_R_Lvalid]
  Right_ReA0/1 -> [Right_ReOp_A0]  "Right_Re"
  Right_LaneA0/1 -> [Right_LaneOp_A0]  "Right_Lane"
  Left_ReA0/1 -> [Left_ReOp_A0]  "Left_Re"
  Left_LaneA0/1 -> [Left_LaneOp_A0]  "Left_Lane"
  Left_ReValid/1 -> [Orginal_L_Revalid]
  Left_LaneValid/1 -> [Orginal_L_Lvalid]
  [Left_else] -> Switch Case Action Subsystem4/Action
  If1/3 -> [Right_else]
  Data Type Conversion5/1 -> If/2
  If/1 -> Switch Case Action Subsystem/Action
  If/2 -> Switch Case Action Subsystem1/Action
  Data Type Conversion6/1 -> If1/1
  Switch Case Action Subsystem/1(Out1) -> Merge/1
  [Right_else] -> Switch Case Action Subsystem5/Action
  [Host_RRE] -> Data Type Conversion7/1
  If/3 -> [Left_else]
  [Host_LRE] -> Data Type Conversion5/1
  Data Type Conversion/1 -> If/1
  Switch Case Action Subsystem2/1(Out1) -> Merge1/1
  If1/2 -> Switch Case Action Subsystem3/Action
  Switch Case Action Subsystem1/1(Out1) -> Merge/2
  Switch Case Action Subsystem3/1(Out1) -> Merge1/2
  [Host_LLane] -> Data Type Conversion/1
  Data Type Conversion7/1 -> If1/2
  Switch Case Action Subsystem4/1(Out1) -> Merge/3
  [Host_RLane] -> Data Type Conversion6/1
  If1/1 -> Switch Case Action Subsystem2/Action
  Switch Case Action Subsystem5/1(Out1) -> Merge1/3
  Compare To Constant4/1 -> Logical Operator24/3
  [Orginal_L_Lvalid] -> Compare To Constant3/1
  Compare To Zero2/1 -> Logical Operator24/1
  [Orginal_L_Lvalid] -> Compare To Constant5/1
  [Left_ReOp_A0] -> Add1/2
  Add1/1 -> Compare To Zero2/1
  [Orginal_L_Revalid] -> Compare To Constant4/1
  Logical Operator29/1 -> Logical Operator25/1
  Logical Operator24/1 -> Logical Operator25/2
  [Left_LaneOp_A0] -> Add4/1
  [Left_ReOp_A0] -> Add4/2
  Add4/1 -> Compare To Zero17/1
  [Orginal_L_Revalid] -> Compare To Constant38/1
  Compare To Zero26/1 -> Logical Operator31/1
  Logical Operator28/1 -> Logical Operator27/1
  [Orginal_L_Revalid] -> Compare To Constant6/1
  [Orginal_L_Lvalid] -> Compare To Constant1/1
  Logical Operator35/1 -> Logical Operator32/1
  Logical Operator30/1 -> Logical Operator27/2
  Compare To Constant2/1 -> Logical Operator28/2
  Logical Operator25/1 -> [Host_LLane]
  [Right_ReOp_A0] -> Add5/2
  [Orginal_L_Revalid] -> Compare To Constant2/1
  Compare To Constant8/1 -> Logical Operator31/2
  Compare To Zero17/1 -> Logical Operator30/1
  Compare To Zero23/1 -> Logical Operator36/1
  Logical Operator27/1 -> [Host_LRE]
  Compare To Constant5/1 -> Logical Operator30/2
  [Left_LaneOp_A0] -> Add1/1
  Compare To Constant1/1 -> Logical Operator29/1
  [Orginal_R_Revalid] -> Compare To Constant10/1
  Compare To Constant10/1 -> Logical Operator34/2
  Compare To Constant12/1 -> Logical Operator36/3
  Compare To Constant11/1 -> Logical Operator36/2
  [Orginal_R_Revalid] -> Compare To Constant9/1
  [Orginal_L_Lvalid] -> Compare To Constant11/1
  [Orginal_R_Lvalid] -> Compare To Constant37/1
  [Right_LaneOp_A0] -> Add6/1
  Logical Operator36/1 -> Logical Operator33/2
  [Right_ReOp_A0] -> Add6/2
  [Orginal_R_Revalid] -> Compare To Constant23/1
  Logical Operator34/1 -> Logical Operator33/1
  [Right_LaneOp_A0] -> Add5/1
  Logical Operator31/1 -> Logical Operator32/2
  [Orginal_R_Lvalid] -> Compare To Constant8/1
  Compare To Constant/1 -> Logical Operator28/1
  Compare To Constant23/1 -> Logical Operator35/2
  Logical Operator32/1 -> [Host_RLane]
  Compare To Constant38/1 -> Logical Operator29/2
  Compare To Constant6/1 -> Logical Operator30/3
  Add6/1 -> Compare To Zero23/1
  Compare To Constant9/1 -> Logical Operator31/3
  [Orginal_L_Revalid] -> Compare To Constant12/1
  Compare To Constant3/1 -> Logical Operator24/2
  [Orginal_R_Lvalid] -> Compare To Constant7/1
  [Orginal_L_Lvalid] -> Compare To Constant/1
  Compare To Constant37/1 -> Logical Operator34/1
  Add5/1 -> Compare To Zero26/1
  Compare To Constant7/1 -> Logical Operator35/1
  Logical Operator33/1 -> [Host_RRE]

== system PvtSubSys_HMI/HMI2.12/IFC_Signal1/Subsystem20 ==
  note: When the vehicle stops, stop updating
  note: 存在一帧丢失状况
  standstill : Inport
  in : Inport  Port=2
  Compare To Constant10 : simulink/Logic and Bit Operations/Compare To Constant  relop===  const=1  OutDataTypeStr=boolean
  Compare To Constant9 : simulink/Logic and Bit Operations/Compare To Constant  relop===  const=0  OutDataTypeStr=boolean
  Logical Operator8 : Logic  AllPortsSameDT=off  OutDataTypeStr=boolean
  MATLAB Function1 : MATLAB Function  TreatAsAtomicUnit=on
  Unit Delay : UnitDelay  SampleTime=-1  HasFrameUpgradeWarning=on
  Unit Delay3 : UnitDelay  SampleTime=-1  HasFrameUpgradeWarning=on
  out : Outport
  wires:
  Logical Operator8/1 -> MATLAB Function1/3(update)
  standstill/1 -> MATLAB Function1/1(standstill), Compare To Constant10/1, Unit Delay3/1
  Compare To Constant9/1 -> Logical Operator8/1
  in/1 -> MATLAB Function1/2(in)
  MATLAB Function1/2(recorder) -> Unit Delay/1
  Unit Delay3/1 -> Compare To Constant9/1
  Compare To Constant10/1 -> Logical Operator8/2
  Unit Delay/1 -> MATLAB Function1/4(inrecorder)
  MATLAB Function1/1(out) -> out/1

== system PvtSubSys_HMI/HMI2.12/IFC_Signal1/Subsystem21 ==
  note: 存在一帧丢失状况
  note: When the vehicle stops, stop updating
  standstill : Inport
  in : Inport  Port=2
  Compare To Constant10 : simulink/Logic and Bit Operations/Compare To Constant  relop===  const=1  OutDataTypeStr=boolean
  Compare To Constant9 : simulink/Logic and Bit Operations/Compare To Constant  relop===  const=0  OutDataTypeStr=boolean
  Logical Operator8 : Logic  AllPortsSameDT=off  OutDataTypeStr=boolean
  MATLAB Function1 : MATLAB Function  TreatAsAtomicUnit=on
  Unit Delay : UnitDelay  SampleTime=-1  HasFrameUpgradeWarning=on
  Unit Delay3 : UnitDelay  SampleTime=-1  HasFrameUpgradeWarning=on
  out : Outport
  wires:
  MATLAB Function1/1(out) -> out/1
  Unit Delay/1 -> MATLAB Function1/4(inrecorder)
  Compare To Constant10/1 -> Logical Operator8/2
  Unit Delay3/1 -> Compare To Constant9/1
  MATLAB Function1/2(recorder) -> Unit Delay/1
  in/1 -> MATLAB Function1/2(in)
  Compare To Constant9/1 -> Logical Operator8/1
  standstill/1 -> Unit Delay3/1, Compare To Constant10/1, MATLAB Function1/1(standstill)
  Logical Operator8/1 -> MATLAB Function1/3(update)

== system PvtSubSys_HMI/HMI2.12/IFC_Signal1/Subsystem22 ==
  note: When the vehicle stops, stop updating
  note: 存在一帧丢失状况
  standstill : Inport
  in : Inport  Port=2
  Compare To Constant10 : simulink/Logic and Bit Operations/Compare To Constant  relop===  const=1  OutDataTypeStr=boolean
  Compare To Constant9 : simulink/Logic and Bit Operations/Compare To Constant  relop===  const=0  OutDataTypeStr=boolean
  Logical Operator8 : Logic  AllPortsSameDT=off  OutDataTypeStr=boolean
  MATLAB Function1 : MATLAB Function  TreatAsAtomicUnit=on
  Unit Delay : UnitDelay  SampleTime=-1  HasFrameUpgradeWarning=on
  Unit Delay3 : UnitDelay  SampleTime=-1  HasFrameUpgradeWarning=on
  out : Outport
  wires:
  Logical Operator8/1 -> MATLAB Function1/3(update)
  standstill/1 -> MATLAB Function1/1(standstill), Compare To Constant10/1, Unit Delay3/1
  Compare To Constant9/1 -> Logical Operator8/1
  in/1 -> MATLAB Function1/2(in)
  MATLAB Function1/2(recorder) -> Unit Delay/1
  Unit Delay3/1 -> Compare To Constant9/1
  Compare To Constant10/1 -> Logical Operator8/2
  Unit Delay/1 -> MATLAB Function1/4(inrecorder)
  MATLAB Function1/1(out) -> out/1

== system PvtSubSys_HMI/HMI2.12/IFC_Signal1/Subsystem23 ==
  note: 存在一帧丢失状况
  note: When the vehicle stops, stop updating
  standstill : Inport
  in : Inport  Port=2
  Compare To Constant10 : simulink/Logic and Bit Operations/Compare To Constant  relop===  const=1  OutDataTypeStr=boolean
  Compare To Constant9 : simulink/Logic and Bit Operations/Compare To Constant  relop===  const=0  OutDataTypeStr=boolean
  Logical Operator8 : Logic  AllPortsSameDT=off  OutDataTypeStr=boolean
  MATLAB Function1 : MATLAB Function  TreatAsAtomicUnit=on
  Unit Delay : UnitDelay  SampleTime=-1  HasFrameUpgradeWarning=on
  Unit Delay3 : UnitDelay  SampleTime=-1  HasFrameUpgradeWarning=on
  out : Outport
  wires:
  MATLAB Function1/1(out) -> out/1
  Unit Delay/1 -> MATLAB Function1/4(inrecorder)
  Compare To Constant10/1 -> Logical Operator8/2
  Unit Delay3/1 -> Compare To Constant9/1
  MATLAB Function1/2(recorder) -> Unit Delay/1
  in/1 -> MATLAB Function1/2(in)
  Compare To Constant9/1 -> Logical Operator8/1
  standstill/1 -> Unit Delay3/1, Compare To Constant10/1, MATLAB Function1/1(standstill)
  Logical Operator8/1 -> MATLAB Function1/3(update)

== system PvtSubSys_HMI/HMI2.12/IFC_Signal1/Subsystem24 ==
  note: When the vehicle stops, stop updating
  note: 存在一帧丢失状况
  standstill : Inport
  in : Inport  Port=2
  Compare To Constant10 : simulink/Logic and Bit Operations/Compare To Constant  relop===  const=1  OutDataTypeStr=boolean
  Compare To Constant9 : simulink/Logic and Bit Operations/Compare To Constant  relop===  const=0  OutDataTypeStr=boolean
  Logical Operator8 : Logic  AllPortsSameDT=off  OutDataTypeStr=boolean
  MATLAB Function1 : MATLAB Function  TreatAsAtomicUnit=on
  Unit Delay : UnitDelay  SampleTime=-1  HasFrameUpgradeWarning=on
  Unit Delay3 : UnitDelay  SampleTime=-1  HasFrameUpgradeWarning=on
  out : Outport
  wires:
  Logical Operator8/1 -> MATLAB Function1/3(update)
  standstill/1 -> MATLAB Function1/1(standstill), Compare To Constant10/1, Unit Delay3/1
  Compare To Constant9/1 -> Logical Operator8/1
  in/1 -> MATLAB Function1/2(in)
  MATLAB Function1/2(recorder) -> Unit Delay/1
  Unit Delay3/1 -> Compare To Constant9/1
  Compare To Constant10/1 -> Logical Operator8/2
  Unit Delay/1 -> MATLAB Function1/4(inrecorder)
  MATLAB Function1/1(out) -> out/1

== system PvtSubSys_HMI/HMI2.12/IFC_Signal1/Subsystem25 ==
  note: 存在一帧丢失状况
  note: When the vehicle stops, stop updating
  standstill : Inport
  in : Inport  Port=2
  Compare To Constant10 : simulink/Logic and Bit Operations/Compare To Constant  relop===  const=1  OutDataTypeStr=boolean
  Compare To Constant9 : simulink/Logic and Bit Operations/Compare To Constant  relop===  const=0  OutDataTypeStr=boolean
  Logical Operator8 : Logic  AllPortsSameDT=off  OutDataTypeStr=boolean
  MATLAB Function1 : MATLAB Function  TreatAsAtomicUnit=on
  Unit Delay : UnitDelay  SampleTime=-1  HasFrameUpgradeWarning=on
  Unit Delay3 : UnitDelay  SampleTime=-1  HasFrameUpgradeWarning=on
  out : Outport
  wires:
  MATLAB Function1/1(out) -> out/1
  Unit Delay/1 -> MATLAB Function1/4(inrecorder)
  Compare To Constant10/1 -> Logical Operator8/2
  Unit Delay3/1 -> Compare To Constant9/1
  MATLAB Function1/2(recorder) -> Unit Delay/1
  in/1 -> MATLAB Function1/2(in)
  Compare To Constant9/1 -> Logical Operator8/1
  standstill/1 -> Unit Delay3/1, Compare To Constant10/1, MATLAB Function1/1(standstill)
  Logical Operator8/1 -> MATLAB Function1/3(update)

== system PvtSubSys_HMI/HMI2.12/IFC_Signal1/Subsystem26 ==
  note: When the vehicle stops, stop updating
  note: 存在一帧丢失状况
  standstill : Inport
  in : Inport  Port=2
  Compare To Constant10 : simulink/Logic and Bit Operations/Compare To Constant  relop===  const=1  OutDataTypeStr=boolean
  Compare To Constant9 : simulink/Logic and Bit Operations/Compare To Constant  relop===  const=0  OutDataTypeStr=boolean
  Logical Operator8 : Logic  AllPortsSameDT=off  OutDataTypeStr=boolean
  MATLAB Function1 : MATLAB Function  TreatAsAtomicUnit=on
  Unit Delay : UnitDelay  SampleTime=-1  HasFrameUpgradeWarning=on
  Unit Delay3 : UnitDelay  SampleTime=-1  HasFrameUpgradeWarning=on
  out : Outport
  wires:
  Logical Operator8/1 -> MATLAB Function1/3(update)
  standstill/1 -> MATLAB Function1/1(standstill), Compare To Constant10/1, Unit Delay3/1
  Compare To Constant9/1 -> Logical Operator8/1
  in/1 -> MATLAB Function1/2(in)
  MATLAB Function1/2(recorder) -> Unit Delay/1
  Unit Delay3/1 -> Compare To Constant9/1
  Compare To Constant10/1 -> Logical Operator8/2
  Unit Delay/1 -> MATLAB Function1/4(inrecorder)
  MATLAB Function1/1(out) -> out/1

== system PvtSubSys_HMI/HMI2.12/IFC_Signal1/Subsystem27 ==
  note: 存在一帧丢失状况
  note: When the vehicle stops, stop updating
  standstill : Inport
  in : Inport  Port=2
  Compare To Constant10 : simulink/Logic and Bit Operations/Compare To Constant  relop===  const=1  OutDataTypeStr=boolean
  Compare To Constant9 : simulink/Logic and Bit Operations/Compare To Constant  relop===  const=0  OutDataTypeStr=boolean
  Logical Operator8 : Logic  AllPortsSameDT=off  OutDataTypeStr=boolean
  MATLAB Function1 : MATLAB Function  TreatAsAtomicUnit=on
  Unit Delay : UnitDelay  SampleTime=-1  HasFrameUpgradeWarning=on
  Unit Delay3 : UnitDelay  SampleTime=-1  HasFrameUpgradeWarning=on
  out : Outport
  wires:
  MATLAB Function1/1(out) -> out/1
  Unit Delay/1 -> MATLAB Function1/4(inrecorder)
  Compare To Constant10/1 -> Logical Operator8/2
  Unit Delay3/1 -> Compare To Constant9/1
  MATLAB Function1/2(recorder) -> Unit Delay/1
  in/1 -> MATLAB Function1/2(in)
  Compare To Constant9/1 -> Logical Operator8/1
  standstill/1 -> Unit Delay3/1, Compare To Constant10/1, MATLAB Function1/1(standstill)
  Logical Operator8/1 -> MATLAB Function1/3(update)

== system PvtSubSys_HMI/HMI2.12/IFC_Signal1/Subsystem28 ==
  note: 存在一帧丢失状况
  note: When the vehicle stops, stop updating
  standstill : Inport
  in : Inport  Port=2
  Compare To Constant10 : simulink/Logic and Bit Operations/Compare To Constant  relop===  const=1  OutDataTypeStr=boolean
  Compare To Constant9 : simulink/Logic and Bit Operations/Compare To Constant  relop===  const=0  OutDataTypeStr=boolean
  Logical Operator8 : Logic  AllPortsSameDT=off  OutDataTypeStr=boolean
  MATLAB Function1 : MATLAB Function  TreatAsAtomicUnit=on
  Unit Delay : UnitDelay  SampleTime=-1  HasFrameUpgradeWarning=on
  Unit Delay3 : UnitDelay  SampleTime=-1  HasFrameUpgradeWarning=on
  out : Outport
  wires:
  MATLAB Function1/1(out) -> out/1
  Unit Delay/1 -> MATLAB Function1/4(inrecorder)
  Compare To Constant10/1 -> Logical Operator8/2
  Unit Delay3/1 -> Compare To Constant9/1
  MATLAB Function1/2(recorder) -> Unit Delay/1
  in/1 -> MATLAB Function1/2(in)
  Compare To Constant9/1 -> Logical Operator8/1
  standstill/1 -> Unit Delay3/1, Compare To Constant10/1, MATLAB Function1/1(standstill)
  Logical Operator8/1 -> MATLAB Function1/3(update)

== system PvtSubSys_HMI/HMI2.12/IFC_Signal1/Subsystem29 ==
  note: When the vehicle stops, stop updating
  note: 存在一帧丢失状况
  standstill : Inport
  in : Inport  Port=2
  Compare To Constant10 : simulink/Logic and Bit Operations/Compare To Constant  relop===  const=1  OutDataTypeStr=boolean
  Compare To Constant9 : simulink/Logic and Bit Operations/Compare To Constant  relop===  const=0  OutDataTypeStr=boolean
  Logical Operator8 : Logic  AllPortsSameDT=off  OutDataTypeStr=boolean
  MATLAB Function1 : MATLAB Function  TreatAsAtomicUnit=on
  Unit Delay : UnitDelay  SampleTime=-1  HasFrameUpgradeWarning=on
  Unit Delay3 : UnitDelay  SampleTime=-1  HasFrameUpgradeWarning=on
  out : Outport
  wires:
  Logical Operator8/1 -> MATLAB Function1/3(update)
  standstill/1 -> MATLAB Function1/1(standstill), Compare To Constant10/1, Unit Delay3/1
  Compare To Constant9/1 -> Logical Operator8/1
  in/1 -> MATLAB Function1/2(in)
  MATLAB Function1/2(recorder) -> Unit Delay/1
  Unit Delay3/1 -> Compare To Constant9/1
  Compare To Constant10/1 -> Logical Operator8/2
  Unit Delay/1 -> MATLAB Function1/4(inrecorder)
  MATLAB Function1/1(out) -> out/1

== system PvtSubSys_HMI/HMI2.12/IFC_Signal1/Subsystem3 ==
  note: When the vehicle stops, stop updating
  note: 存在一帧丢失状况
  standstill : Inport
  in : Inport  Port=2
  Compare To Constant10 : simulink/Logic and Bit Operations/Compare To Constant  relop===  const=1  OutDataTypeStr=boolean
  Compare To Constant9 : simulink/Logic and Bit Operations/Compare To Constant  relop===  const=0  OutDataTypeStr=boolean
  Logical Operator8 : Logic  AllPortsSameDT=off  OutDataTypeStr=boolean
  MATLAB Function1 : MATLAB Function  TreatAsAtomicUnit=on
  Unit Delay : UnitDelay  SampleTime=-1  HasFrameUpgradeWarning=on
  Unit Delay3 : UnitDelay  SampleTime=-1  HasFrameUpgradeWarning=on
  out : Outport
  wires:
  Logical Operator8/1 -> MATLAB Function1/3(update)
  standstill/1 -> MATLAB Function1/1(standstill), Compare To Constant10/1, Unit Delay3/1
  Compare To Constant9/1 -> Logical Operator8/1
  in/1 -> MATLAB Function1/2(in)
  MATLAB Function1/2(recorder) -> Unit Delay/1
  Unit Delay3/1 -> Compare To Constant9/1
  Compare To Constant10/1 -> Logical Operator8/2
  Unit Delay/1 -> MATLAB Function1/4(inrecorder)
  MATLAB Function1/1(out) -> out/1
